simulink model "Multilevel"  (R2019a)
settings: Solver=ode45  StartTime=0.0  StopTime=0.2  MaxStep=1e-4  RelTol=1e-3
values from neighbouring files (symbols this model uses):
  alpha_mul_1 = alphas2_sorted(1)    [inputs.m]
  alpha_mul_2 = alphas2_sorted(2)    [inputs.m]
  alpha_mul_3 = alphas2_sorted(3)    [inputs.m]
  f = 50    [inputs.m]
  L = 33e-3    (= 0.033)    [inputs.m]
  R = 33    [inputs.m]
  Vdc = 100    [inputs.m]
libraries: powerlib x25
settings Model: Creator=omar_  LastModifiedBy=omar_
settings DataIOCC: ReturnWorkspaceOutputs=off

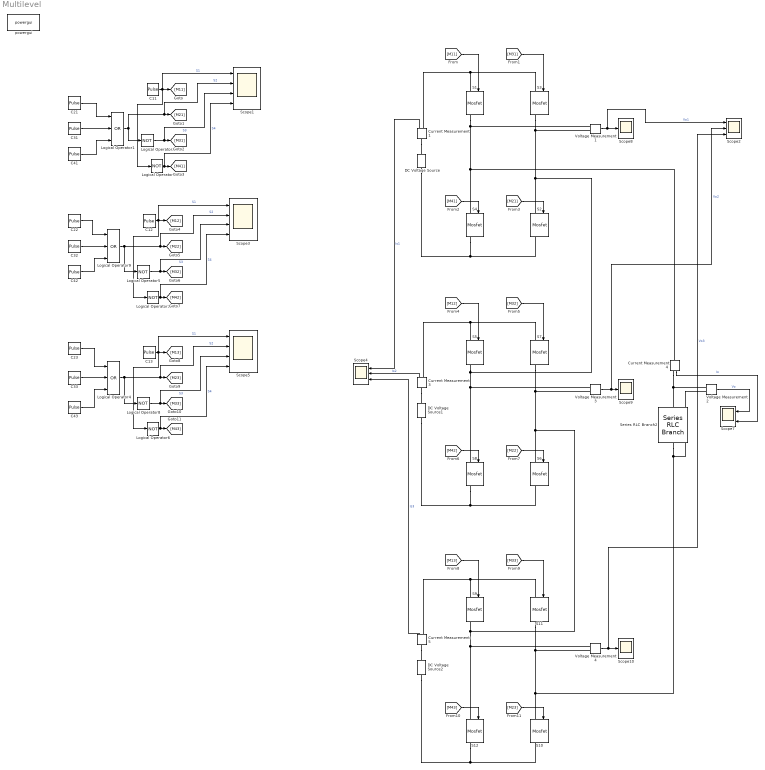
== system Multilevel ==
  C11 : DiscretePulseGenerator  PulseType=Time based  Period=1/f  PulseWidth=50
  C12 : DiscretePulseGenerator  PulseType=Time based  Period=1/f  PulseWidth=50
  C13 : DiscretePulseGenerator  PulseType=Time based  Period=1/f  PulseWidth=50
  C21 : DiscretePulseGenerator  PulseType=Time based  Period=1/f  PulseWidth=((180-(2*alpha_mul_1))/(360))*100  PhaseDelay=(alpha_mul_1/180)/100
  C22 : DiscretePulseGenerator  PulseType=Time based  Period=1/f  PulseWidth=((180-(2*alpha_mul_2))/(360))*100  PhaseDelay=(alpha_mul_2/180)/100
  C23 : DiscretePulseGenerator  PulseType=Time based  Period=1/f  PulseWidth=((180-(2*alpha_mul_3))/(360))*100  PhaseDelay=(alpha_mul_3/180)/100
  C31 : DiscretePulseGenerator  PulseType=Time based  Period=1/f  PulseWidth=((alpha_mul_1)/(360))*100  PhaseDelay=((360-alpha_mul_1)/180)/100
  C32 : DiscretePulseGenerator  PulseType=Time based  Period=1/f  PulseWidth=((alpha_mul_2)/(360))*100  PhaseDelay=((360-alpha_mul_2)/180)/100
  C33 : DiscretePulseGenerator  PulseType=Time based  Period=1/f  PulseWidth=((alpha_mul_3)/(360))*100  PhaseDelay=((360-alpha_mul_3)/180)/100
  C41 : DiscretePulseGenerator  PulseType=Time based  Period=1/f  PulseWidth=((alpha_mul_1)/(360))*100  PhaseDelay=1/100
  C42 : DiscretePulseGenerator  PulseType=Time based  Period=1/f  PulseWidth=((alpha_mul_2)/(360))*100  PhaseDelay=1/100
  C43 : DiscretePulseGenerator  PulseType=Time based  Period=1/f  PulseWidth=((alpha_mul_3)/(360))*100  PhaseDelay=1/100
  Current Measurement{1,3..5} (4 alike) : powerlib/Measurements/Current Measurement  PhasorSimulation=off  OutputType=Magnitude  PSBequivalent=0
      settings: SourceProductName=Simscape Electrical
  DC Voltage Source : powerlib/Electrical Sources/DC Voltage Source  Amplitude=Vdc/3  Measurements=None
      settings: SourceProductName=Simscape Electrical
  DC Voltage Source1 : powerlib/Electrical Sources/DC Voltage Source  Amplitude=Vdc/3  Measurements=None
      settings: SourceProductName=Simscape Electrical
  DC Voltage Source2 : powerlib/Electrical Sources/DC Voltage Source  Amplitude=Vdc/3  Measurements=None
      settings: SourceProductName=Simscape Electrical
  Logical Operator{,2..3,5..6,8} (6 alike) : Logic  Operator=NOT  AllPortsSameDT=off  OutDataTypeStr=boolean
  Logical Operator1 : Logic  Operator=OR  Inputs=3  AllPortsSameDT=off  OutDataTypeStr=boolean
  Logical Operator4 : Logic  Operator=OR  Inputs=3  AllPortsSameDT=off  OutDataTypeStr=boolean
  Logical Operator9 : Logic  Operator=OR  Inputs=3  AllPortsSameDT=off  OutDataTypeStr=boolean
  S{1..12} (12 alike) : powerlib/Power Electronics/Mosfet  Ron=0.1  Lon=0  Rd=0.01  Vfd=0  IC=0  Rs=1e5  Cs=inf  Measurements=on
      settings: SourceProductName=Simscape Electrical
  Scope1 : Scope  NumInputPorts=4
  Scope10 : Scope
  Scope2 : Scope  NumInputPorts=3
  Scope3 : Scope  NumInputPorts=4
  Scope4 : Scope  NumInputPorts=3
  Scope5 : Scope  NumInputPorts=4
  Scope7 : Scope  NumInputPorts=2
  Scope8 : Scope
  Scope9 : Scope
  Series RLC Branch2 : powerlib/Elements/Series RLC Branch  LConnTagsString=__new0  RConnTagsString=__new0  BranchType=RL  Resistance=R  Inductance=L  SetiL0=off  InitialCurrent=0  Capacitance=1e-6  Setx0=off  InitialVoltage=0  Measurements=None
      settings: SourceProductName=Simscape Electrical
  Voltage Measurement{1..4} (4 alike) : powerlib/Measurements/Voltage Measurement  PhasorSimulation=off  OutputType=Magnitude  PSBequivalent=0
      settings: SourceProductName=Simscape Electrical
  powergui : powerlib/powergui  Priority=1  SimulationMode=Continuous  SampleTime=1e-6  frequency=60  Iterations=50  frequencyindice=0  Pbase=100e6  ErrMax=1e-4  UnitsV=kV  UnitsW=MW  buscounter=0  FunctionMessages=off  echomessages=off  EnableUseOfTLC=off  CurrentSourceSwitches=off  DisableSnubberDevices=off  DisableRonSwitches=off  DisableVfSwitches=off  DisplayEquations=off  AutomaticDiscreteSolvers=off  SolverType=Tustin/Backward Euler (TBE)  Interpol=off  ExternalGateDelay=off  methode=off  Ts=100  x0status=blocks  SPID=on  SwTol=0  HookPort=off  NonlinearTolerance=0  nMaxIteration=15  ContinueOnMaxIteration=off  RestoreLinks=warning  ResistiveCurrentMeasurement=off  Frange=[0:2:500]  Ylog=off  Xlog=on  ShowGrid=off  save=off  variable=ZData  structure=Outputs  ZoomFFT=off  StartTime=0.08  cycles=3  DisplayStyle=2  fundamental=50  FreqAxis=off  MaxFrequency=1000  frequencyindicesteady=1  RmsSteady=1  display=off
      settings: SourceProductName=Simscape Electrical
  wires:
  [M41] -> S4/1
  [M21] -> S2/1
  [M11] -> S1/1
  [M31] -> S3/1
  Logical Operator2/1 -> Scope1/3, [M31]  "S3"
  C11/1 -> Logical Operator/1, [M11], Scope1/1  "S1"
  [M12] -> S5/1
  [M22] -> S6/1
  Current Measurement3/1 -> Scope4/2  "Is2"
  [M42] -> S8/1
  [M32] -> S7/1
  Voltage Measurement2/1 -> Scope7/1  "Vo"
  Current Measurement4/1 -> Scope7/2  "Io"
  [M13] -> S9/1
  [M23] -> S10/1
  [M43] -> S12/1
  [M33] -> S11/1
  Voltage Measurement1/1 -> Scope2/1, Scope8/1  "Vo1"
  Voltage Measurement3/1 -> Scope2/2, Scope9/1  "Vo2"
  Voltage Measurement4/1 -> Scope2/3, Scope10/1  "Vo3"
  Logical Operator/1 -> Scope1/4, [M41]  "S4"
  C21/1 -> Logical Operator1/1
  C31/1 -> Logical Operator1/2
  Logical Operator1/1 -> Scope1/2, [M21], Logical Operator2/1  "S2"
  C12/1 -> Logical Operator3/1, [M12], Scope3/1  "S1"
  Logical Operator9/1 -> Logical Operator5/1, Scope3/2, [M22]  "S2"
  Logical Operator3/1 -> Scope3/4, [M42]  "S4"
  Logical Operator5/1 -> Scope3/3, [M32]  "S3"
  C13/1 -> Logical Operator6/1, [M13], Scope5/1  "S1"
  Logical Operator4/1 -> Logical Operator8/1, Scope5/2, [M23]  "S2"
  Logical Operator6/1 -> Scope5/4, [M43]  "S4"
  Logical Operator8/1 -> Scope5/3, [M33]  "S3"
  C41/1 -> Logical Operator1/3
  C23/1 -> Logical Operator4/1
  C33/1 -> Logical Operator4/2
  C32/1 -> Logical Operator9/2
  C22/1 -> Logical Operator9/1
  C42/1 -> Logical Operator9/3
  C43/1 -> Logical Operator4/3
  Current Measurement5/1 -> Scope4/3  "Is3"
  Current Measurement1/1 -> Scope4/1  "Is1"
  connections:
  S1/RConn1 -- Voltage Measurement1/LConn1 -- Current Measurement4/LConn1 -- S4/LConn1
  Current Measurement1/RConn1 -- S3/LConn1 -- S1/LConn1
  Voltage Measurement1/LConn2 -- S3/RConn1 -- S2/LConn1 -- Voltage Measurement3/LConn1 -- S8/LConn1 -- S5/RConn1
  S4/RConn1 -- S2/RConn1 -- DC Voltage Source/LConn1
  Current Measurement1/LConn1 -- DC Voltage Source/RConn1
  S8/RConn1 -- S6/RConn1 -- DC Voltage Source1/LConn1
  Current Measurement3/RConn1 -- S7/LConn1 -- S5/LConn1
  Current Measurement3/LConn1 -- DC Voltage Source1/RConn1
  S12/RConn1 -- S10/RConn1 -- DC Voltage Source2/LConn1
  Voltage Measurement2/LConn1 -- Current Measurement4/RConn1 -- Series RLC Branch2/LConn1
  Current Measurement5/RConn1 -- S11/LConn1 -- S9/LConn1
  Current Measurement5/LConn1 -- DC Voltage Source2/RConn1
  S7/RConn1 -- Voltage Measurement3/LConn2 -- S6/LConn1 -- S12/LConn1 -- Voltage Measurement4/LConn1 -- S9/RConn1
  S11/RConn1 -- Voltage Measurement2/LConn2 -- Series RLC Branch2/RConn1 -- S10/LConn1 -- Voltage Measurement4/LConn2
